simulink model "two_system_model"  (R2024a)
settings: Solver=VariableStepAuto  StartTime=0.0  StopTime=10.0  MaxStep=0.1  RelTol=1e-3
settings Model: Creator=Abbas  LastModifiedBy=Abbas

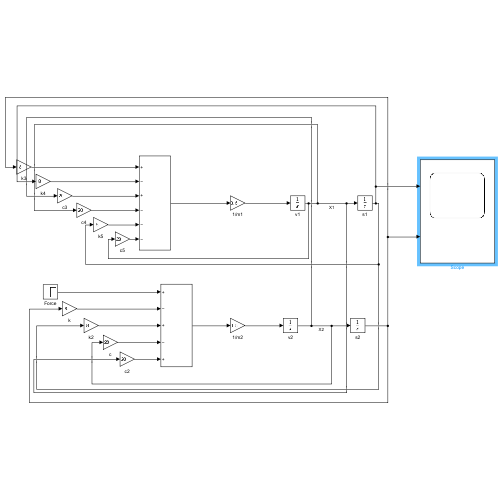
[thumbnail: Simulink's stored preview of the top-level diagram]
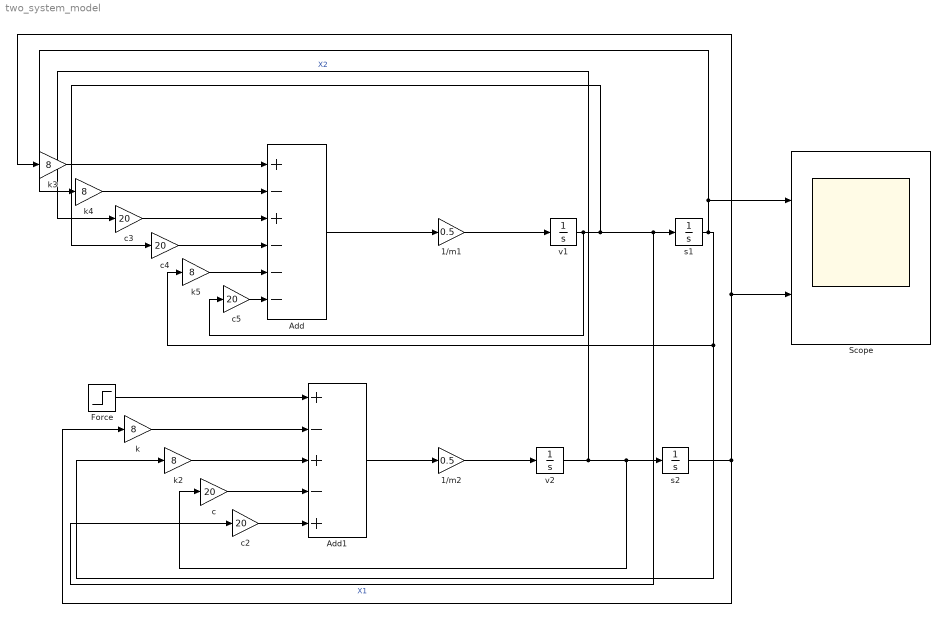
== system two_system_model ==
  1/m1 : Gain  Gain=0.5
  1/m2 : Gain  Gain=0.5
  Add : Sum  Inputs=+-+---
  Add1 : Sum  Inputs=+-+-+
  Force : Step  SampleTime=0
  Scope : Scope  NumInputPorts=2
  c{,2..5} (5 alike) : Gain  Gain=20
  k{,2..5} (5 alike) : Gain  Gain=8
  s1 : Integrator  InitialCondition=0.1
  s2 : Integrator  InitialCondition=0.1
  v1 : Integrator  InitialCondition=10
  v2 : Integrator  InitialCondition=10
  wires:
  v1/1 -> c4/1, c2/1, s1/1, c5/1  "X1"
  v2/1 -> c3/1, c/1, s2/1  "X2"
  Add1/1 -> 1/m2/1
  1/m2/1 -> v2/1
  k/1 -> Add1/2
  k2/1 -> Add1/3
  c/1 -> Add1/4
  c2/1 -> Add1/5
  s2/1 -> Scope/2, k3/1, k/1
  s1/1 -> k4/1, Scope/1, k5/1, k2/1
  1/m1/1 -> v1/1
  Add/1 -> 1/m1/1
  k3/1 -> Add/1
  k4/1 -> Add/2
  c3/1 -> Add/3
  c4/1 -> Add/4
  k5/1 -> Add/5
  c5/1 -> Add/6
  Force/1 -> Add1/1
